simulink model "boat_pp_diff"  (R2025b)
settings: Solver=ode3  StartTime=0.0  StopTime=200.0  FixedStep=0.02  RelTol=1e-3
values from neighbouring files (symbols this model uses):
  deadband = 0.05    [init_boat.m]
  kou = 1.6 / omegamax    (= 0.4)    [init_boat.m]
  kvu = 1.0 / vmax    (= 0.833333333333)    [init_boat.m]
  psi0 = atan2(W(2,2)-W(1,2), W(2,1)-W(1,1))    [init_boat.m]
  tau_m = 0.10    (= 0.1)    [init_boat.m]
  Ts = 0.02    [init_boat.m]
  v_cx = 0.00    (= 0)    [init_boat.m]
  v_cy = 0.10    (= 0.1)    [init_boat.m]
  vmax = 1.2    [init_boat.m]
  W = m_snake_coverage(5.0, 2.0,          'LaneSpacing', 0.25,          'Margin',      0.10,          'TurnRadius',  0.125,          'ds',          0.05)    [init_boat.m]    (also in m_lattice_pool_nav.m = densify_xy(xy, 0.1); m_snake_coverage.m = [W; [repmat(xb(end),numel(y_conn),1) y_conn(:)]])
  x0 = W(1,1)    [init_boat.m]
  y0 = W(1,2)    [init_boat.m]
undefined symbols (not defined in the file or in its folder): dspblkCoreblockFVToolHelper, gcbh, wrench
libraries: ros2lib x3, robotcorelib x1, robotmobilelib x1, robotalgslib x1
settings Model: Creator=larsd  LastModifiedBy=larsd

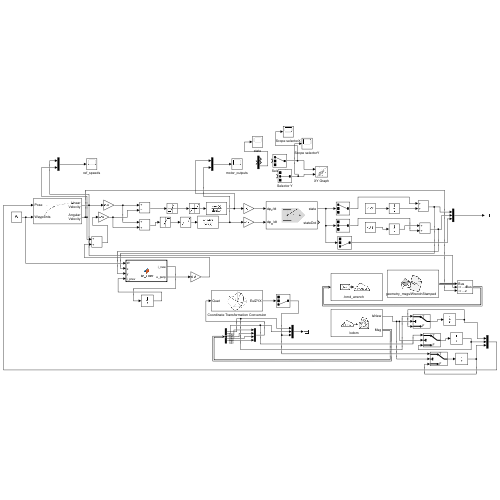
[thumbnail: Simulink's stored preview of the top-level diagram]
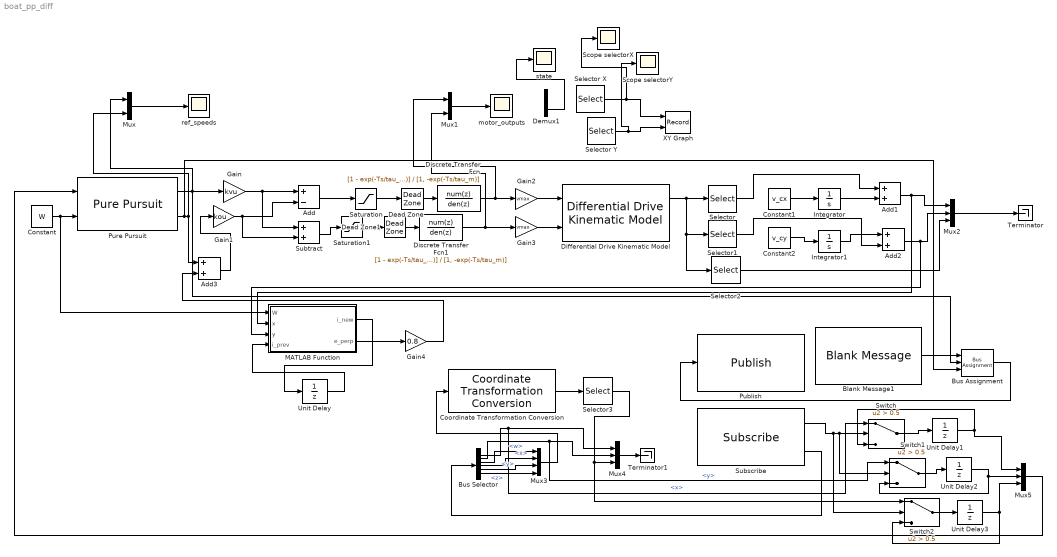
== system boat_pp_diff ==
  Add : Sum  Inputs=+-
  Add1 : Sum
  Add2 : Sum
  Add3 : Sum
  Blank Message1 : ros2lib/Blank Message  messageClass=Message  entityType=geometry_msgs/WrenchStamped  messageType=geometry_msgs/WrenchStamped  SampleTime=inf
  Bus Assignment : BusAssignment  AssignedSignals=wrench.force.x,wrench.torque.z
  Bus Selector : BusSelector  OutputSignals=pose.pose.position.x,pose.pose.position.y,pose.pose.orientation.w,pose.pose.orientation.x,pose.pose.orientation.y,pose.pose.orientation.z
  Constant : Constant  Value=W  SampleTime=-1
  Constant1 : Constant  Value=v_cx
  Constant2 : Constant  Value=v_cy
  Coordinate Transformation Conversion : robotcorelib/Coordinate Transformation Conversion  InputRepresentation=Quaternion  InputEulerSequence=ZYX  ShowTrVecInputPort=on  OutputRepresentation=Euler Angles  OutputEulerSequence=ZYX  ShowTrVecOutputPort=on  SimulateUsing=Interpreted execution
  Dead Zone : DeadZone  LowerValue=-deadband  UpperValue=deadband
  Dead Zone1 : DeadZone  LowerValue=-deadband  UpperValue=deadband
  Demux1 : Demux  Outputs=3
  Differential Drive Kinematic Model : robotmobilelib/Differential Drive Kinematic Model  VehicleInputs=Wheel Speeds  WheelRadius=1  WheelSpeedRange=[-inf inf]  TrackWidth=b  InitialState=[x0; y0; psi0]  SimulateUsing=Interpreted execution
  Discrete Transfer Fcn : DiscreteTransferFcn  LoadFcn=dspblkCoreblockFVToolHelper(gcbh,'load');  Numerator=[1 - exp(-Ts/tau_m)]  Denominator=[1, -exp(-Ts/tau_m)]
      settings: CopyFcn=dspblkCoreblockFVToolHelper(gcbh,'copy');  DeleteFcn=dspblkCoreblockFVToolHelper(gcbh,'close');  ModelCloseFcn=dspblkCoreblockFVToolHelper(gcbh,'close');  PreSaveFcn=dspblkCoreblockFVToolHelper(gcbh,'presave');  PostSaveFcn=dspblkCoreblockFVToolHelper(gcbh,'postsave');  CloseFcn=dspblkCoreblockFVToolHelper(gcbh,'close');
  Discrete Transfer Fcn1 : DiscreteTransferFcn  LoadFcn=dspblkCoreblockFVToolHelper(gcbh,'load');  Numerator=[1 - exp(-Ts/tau_m)]  Denominator=[1, -exp(-Ts/tau_m)]
      settings: CopyFcn=dspblkCoreblockFVToolHelper(gcbh,'copy');  DeleteFcn=dspblkCoreblockFVToolHelper(gcbh,'close');  ModelCloseFcn=dspblkCoreblockFVToolHelper(gcbh,'close');  PreSaveFcn=dspblkCoreblockFVToolHelper(gcbh,'presave');  PostSaveFcn=dspblkCoreblockFVToolHelper(gcbh,'postsave');  CloseFcn=dspblkCoreblockFVToolHelper(gcbh,'close');
  Gain : Gain  Gain=kvu
  Gain1 : Gain  Gain=kou
  Gain2 : Gain  Gain=vmax
  Gain3 : Gain  Gain=vmax
  Gain4 : Gain  Gain=0.8
  Integrator : Integrator
  Integrator1 : Integrator
  MATLAB Function : MATLAB Function  TreatAsAtomicUnit=on
  Mux : Mux  Inputs=2
  Mux1 : Mux  Inputs=2
  Mux2 : Mux  Inputs=3
  Mux3 : Mux
  Mux4 : Mux  Inputs=3
  Mux5 : Mux  Inputs=3
  Publish : ros2lib/Publish  topicSource=Specify your own  topic=/cmd_wrench  messageType=geometry_msgs/WrenchStamped  QOSHistory=Keep last  QOSDepth=10  QOSReliability=Reliable  QOSDurability=Volatile  QOSDeadline=Inf  QOSLifespan=Inf  QOSLiveliness=Automatic  QOSLeaseDuration=Inf  QOSAvoidROSNamespaceConventions=off
  Pure Pursuit : robotalgslib/Pure Pursuit  DesiredLinearVelocityPort=off  DesiredLinearVelocity=v_des  MaxAngularVelocity=omega_max  LookaheadDistancePort=off  LookaheadDistance=lookahead  TargetDirPort=off  SimulateUsing=Code generation
      settings: LibrarySourceBlock=navlib/Control Algorithms/Pure Pursuit
  Saturation : Saturate  UpperLimit=1  LowerLimit=-1
  Saturation1 : Saturate  UpperLimit=1  LowerLimit=-1
  Scope selectorX : Scope
      settings: ActiveDisplayYMinimum=-37.844230218102112  ActiveDisplayYMaximum=16.6968282622902
  Scope selectorY : Scope
      settings: ActiveDisplayYMinimum=-39.044864820032323  ActiveDisplayYMaximum=4.3383183133369236
  Selector : Selector  InputPortWidth=3  IndexOptions=Index vector (dialog)  Indices=[1]  OutputSizes=1
  Selector X : Selector  InputPortWidth=3  IndexOptions=Index vector (dialog)  Indices=[1]  OutputSizes=1
  Selector Y : Selector  InputPortWidth=3  IndexOptions=Index vector (dialog)  Indices=[2]  OutputSizes=1
  Selector1 : Selector  InputPortWidth=3  IndexOptions=Index vector (dialog)  Indices=[2]  OutputSizes=1
  Selector2 : Selector  InputPortWidth=3  IndexOptions=Index vector (dialog)  Indices=[3]  OutputSizes=1
  Selector3 : Selector  InputPortWidth=3  IndexOptions=Index vector (dialog)  Indices=[3]  OutputSizes=1
  Subscribe : ros2lib/Subscribe  topicSource=Specify your own  topic=/odom  messageType=nav_msgs/Odometry  sampleTime=0.02  QOSHistory=Keep last  QOSDepth=10  QOSReliability=Reliable  QOSDurability=Volatile  QOSDeadline=Inf  QOSLifespan=Inf  QOSLiveliness=Automatic  QOSLeaseDuration=Inf  QOSAvoidROSNamespaceConventions=off
  Subtract : Sum
  Switch : Switch  Criteria=u2 > Threshold  Threshold=0.5  SaturateOnIntegerOverflow=off  InputSameDT=off
  Switch1 : Switch  Criteria=u2 > Threshold  Threshold=0.5  SaturateOnIntegerOverflow=off  InputSameDT=off
  Switch2 : Switch  Criteria=u2 > Threshold  Threshold=0.5  SaturateOnIntegerOverflow=off  InputSameDT=off
  Terminator : Terminator
  Terminator1 : Terminator
  Unit Delay{,1..3} (4 alike) : UnitDelay  SampleTime=-1  HasFrameUpgradeWarning=on
  XY Graph : Record  NumPorts=2.0  FileSettingsInternal="{\"entries\":[{\"content\":{\"excelSettings\":{\"content\":{},\"type\":\"Streamout.ExcelSettings\"},\"parquetSettings\":{\"content\":{},\"type\":\"Streamout.ParquetSettings\"}},\"type\":\"Streamout.FileSettingStorage\",\"uuid\":\"\"}],\"packageUris\":[\"http:\\/\\/schema.mathworks.com\\/mf0\\/streamout_blocks\\/R2020a\"],\"version\":\"1.0\"}"  FrameSettings=[0, 0]  Layout=[1 1]  SignalsInternal="{\"entries\":[{\"content\":{\"signals\":[{\"content\":{\"blockPath\":[],\"dimensions\":[1],\"domain\":\"\",\"lineColor\":\"#a2142f\",\"lineWidth\":2,\"plots\":[ 1 ],\"port\":1,\"signalID\":1,\"signalName\":\"Selector X\"},\"type\":\"RecordBlkView.Signal\",\"uuid\":\"\"},{\"content\":{\"blockPath\":[],\"dimensions\":[1],\"domain\":\"\",\"lineColor\":\"#139fff\",\"plots\":[ 1 ],\"port\":2,\"signalID\":2,\"signalName\":\"Selector Y\"},\"type\":\"RecordBlkView.Signal\",\"uuid\":\"\"}]},\"type\":\"RecordBlkView.InputSignals\",\"uuid\":\"\"}],\"packageUris\":[\"http:\\/\\/schema.mathworks.com\\/mf0\\/streamout_blocks\\/R2020a\"],\"version\":\"1.0\"}"  VisualizationBindings="{\"xyplotplugin\":{\"info\":[{\"series\":[{\"bindingParametersList\":[{\"parameter\":\"X-Axis\",\"signalID\":1,\"signalName\":\"Selector X\"},{\"parameter\":\"Y-Axis\",\"signalID\":2,\"signalName\":\"Selector Y\"}],\"seriesID\":0}],\"subplotID\":1}]}}"  CompatibilityTag=XY
  motor_outputs : Scope
      settings: ActiveDisplayYMinimum=-0.42940207734180436  ActiveDisplayYMaximum=0.799848525879461  DataLoggingMaxPoints=2000  DataLoggingDecimation=5  DataLoggingVariableName=motor
  ref_speeds : Scope
      settings: ActiveDisplayYMinimum=-0.65928176375190983  ActiveDisplayYMaximum=1.4289416292492949  DataLoggingMaxPoints=2000  DataLoggingDecimation=5  DataLoggingVariableName=speeds
  state : Scope
      settings: ActiveDisplayYMinimum=-7.4267826408666524  ActiveDisplayYMaximum=8.2044170335993272  DataLoggingMaxPoints=2000  DataLoggingDecimation=5  DataLoggingVariableName=state
  wires:
  Constant/1 -> MATLAB Function/1(W), Pure Pursuit/2
  Pure Pursuit/1 -> Bus Assignment/2, Gain/1, Mux/1
  Gain/1 -> Subtract/1, Add/1
  Gain1/1 -> Subtract/2, Add/2
  Subtract/1 -> Saturation1/1
  Add/1 -> Saturation/1
  Saturation/1 -> Dead Zone/1
  Saturation1/1 -> Dead Zone1/1
  Dead Zone/1 -> Discrete Transfer Fcn/1
  Dead Zone1/1 -> Discrete Transfer Fcn1/1
  Discrete Transfer Fcn/1 -> Mux1/1, Gain2/1
  Discrete Transfer Fcn1/1 -> Mux1/2, Gain3/1
  Gain2/1 -> Differential Drive Kinematic Model/1
  Gain3/1 -> Differential Drive Kinematic Model/2
  Mux/1 -> ref_speeds/1
  Mux1/1 -> motor_outputs/1
  Demux1/3 -> state/1
  Selector X/1 -> Scope selectorX/1, XY Graph/1
  Selector Y/1 -> Scope selectorY/1, XY Graph/2
  Differential Drive Kinematic Model/1 -> Selector2/1, Selector1/1, Selector/1
  Constant1/1 -> Integrator/1
  Constant2/1 -> Integrator1/1
  Integrator/1 -> Add1/2
  Selector/1 -> Add1/1
  Selector1/1 -> Add2/2
  Integrator1/1 -> Add2/1
  Add1/1 -> MATLAB Function/2(x), Mux2/1
  Add2/1 -> MATLAB Function/3(y), Mux2/2
  Selector2/1 -> Mux2/3
  MATLAB Function/1(i_new) -> Unit Delay/1
  Unit Delay/1 -> MATLAB Function/4(i_prev)
  MATLAB Function/2(e_perp) -> Gain4/1
  Pure Pursuit/2 -> Bus Assignment/3, Mux/2, Add3/1
  Gain4/1 -> Add3/2
  Add3/1 -> Gain1/1
  Subscribe/2 -> Bus Selector/1
  Bus Selector/6 -> Mux3/4  "<z>"
  Bus Selector/5 -> Mux3/3  "<y>"
  Bus Selector/4 -> Mux3/2  "<x>"
  Bus Selector/3 -> Mux3/1  "<w>"
  Mux3/1 -> Coordinate Transformation Conversion/1
  Coordinate Transformation Conversion/1 -> Selector3/1
  Bus Selector/2 -> Switch1/1, Mux4/2  "<y>"
  Bus Selector/1 -> Switch/1, Mux4/1  "<x>"
  Selector3/1 -> Switch2/1, Mux4/3
  Mux2/1 -> Terminator/1
  Bus Assignment/1 -> Publish/1
  Blank Message1/1 -> Bus Assignment/1
  Subscribe/1 -> Switch2/2, Switch1/2, Switch/2
  Switch2/1 -> Unit Delay3/1
  Switch1/1 -> Unit Delay2/1
  Switch/1 -> Unit Delay1/1
  Unit Delay1/1 -> Mux5/1, Switch/3
  Unit Delay2/1 -> Mux5/2, Switch1/3
  Unit Delay3/1 -> Mux5/3, Switch2/3
  Mux5/1 -> Pure Pursuit/1
  Mux4/1 -> Terminator1/1

== matlab function boat_pp_diff/MATLAB Function ==
  data: i_new output; W input; e_perp output; x input; y input; i_prev input
function [i_new, e_perp] = cte_error(W, x, y, i_prev)
% W (Nx2): waypoints i meter
% (x,y):   posisjon i meter
% i_prev:  indeks for forrige aktive linjesegment (1..N-1)

N = size(W,1);
if N < 2
    i_new = 1; e_perp = 0; return;
end

% ---- begrens søkeområdet så vi slipper å skanne hele W hver gang
i0 = max(1, i_prev-2);
i1 = min(N-1, i_prev+2);

best_d2 = inf;
i_best  = i_prev;
e_best  = 0;

p = [x y];

for k = i0:i1
    P = W(k,:);  Q = W(k+1,:);
    t = Q - P;   L2 = t(1)^2 + t(2)^2;
    if L2 < 1e-12, continue; end

    % projisering av p på segment k
    s = dot(p-P, t) / L2;          % uparametrisert posisjon langs segment
    s = min(max(s,0),1);           % clamp innen segmentet
    C = P + s*t;                   % nærmeste punkt på segmentet
    r = p - C;
    d2 = r(1)^2 + r(2)^2;

    % SIGNERT tverrfeil (venstre = positiv ift. segmentretning)
    n = [ -t(2)  t(1) ];           % normal til t
    e = (n(1)*r(1) + n(2)*r(2)) / sqrt(L2);

    if d2 < best_d2
        best_d2 = d2;  i_best = k;  e_best = e;
    end
end

i_new = i_best;
e_perp = e_best;
